simulink model "SIM_EXO_DAL_MN"  (R2021b)
settings: Solver=VariableStepAuto  StartTime=0.0  StopTime=60  FixedStep=0.0001  RelTol=1e-4
undefined symbols (not defined in the file): b, dq, q, X, Y, Z
libraries: sm_lib x47, nesl_utility x7
(part 20 of 24)

== matlab function SIM_EXO_DAL_MN/PD+g(DIN)/Gq ==
  data: q input; G output
function G = Gq(q)
%#codegen
q1 = q(1);
q2 = q(2);
q3 = q(3);
q4 = q(4);
q5 = q(5);
q6 = q(6);
%    This function was generated by the Symbolic Math Toolbox version 9.0.
%    02-Dec-2021 21:38:44

t2 = cos(q4);
t3 = cos(q5);
t4 = cos(q6);
t5 = sin(q4);
t6 = sin(q5);
t7 = sin(q6);
t8 = q1+q2;
t16 = 9.007199254740992e+15;
t9 = cos(t8);
t10 = sin(t8);
t19 = (q3.*t16)./9.007199254740992e+15;
t11 = t10.*7.742227997977903e+15;
t12 = t9.*4.602992943936994e+15;
t13 = t10.*4.602992943936994e+15;
t14 = t9.*7.742227997977903e+15;
t20 = cos(t19);
t21 = sin(t19);
t22 = t3.*t10.*1.11711378834605e-4;
t23 = t3.*t9.*1.878983903386652e-4;
t25 = t5.*t6.*t10.*1.878983903386652e-4;
t26 = t5.*t6.*t9.*3.16044842165395e-4;
t31 = t10.*3.412222012061753e-3;
t32 = t9.*5.313226374396773e-3;
t15 = -t13;
t17 = t11+t12;
t24 = -t22;
t27 = -t26;
t28 = t20.*7.38843356682345e-1;
t29 = t20.*2.61156643317655e-1;
t30 = t20.*4.392651260556773e-1;
t33 = -t31;
t34 = t20.*t23;
t35 = t3.*t10.*t20.*3.16044842165395e-4;
t36 = t3.*t9.*t20.*(-1.878983903386652e-4);
t38 = t5.*t6.*t9.*t20.*1.11711378834605e-4;
t39 = t20.*t25;
t41 = t5.*t6.*t10.*t20.*(-1.878983903386652e-4);
t44 = t2.*t16.*t21.*(t13-t14).*(-1.232595164407831e-32);
t46 = t5.*t16.*t21.*(t13-t14).*(-1.232595164407831e-32);
t47 = (t5.*t16.*t21.*(t13-t14))./8.112963841460668e+31;
t48 = t2.*t6.*t10.*t16.*t21.*4.082091644006594e-20;
t49 = t2.*t6.*t9.*t16.*t21.*2.426929178367519e-20;
t55 = t9.*t20.*1.796561051029836e-3;
t56 = t10.*t20.*3.021813293822463e-3;
t18 = t14+t15;
t37 = -t35;
t40 = -t38;
t42 = (t2.*t16.*t17.*t21)./8.112963841460668e+31;
t43 = (t5.*t16.*t17.*t21)./8.112963841460668e+31;
t50 = -t48;
t51 = -t49;
t52 = t28+2.61156643317655e-1;
t53 = t29+7.38843356682345e-1;
t54 = t30-4.392651260556773e-1;
t57 = -t55;
t58 = -t56;
t45 = -t43;
t59 = t9.*t52;
t60 = t9.*t53;
t61 = t10.*t52;
t62 = t10.*t53;
t63 = t9.*t54;
t64 = t10.*t54;
t65 = -t62;
t66 = -t64;
t67 = t61+t63;
t68 = t60+t64;
t74 = -t2.*(t62-t63);
t76 = -t5.*(t62-t63);
t84 = -t3.*(t5.*(t62-t63)+(t2.*t16.*t21.*(t13-t14))./8.112963841460668e+31);
t85 = -t6.*(t5.*(t62-t63)+(t2.*t16.*t21.*(t13-t14))./8.112963841460668e+31);
t86 = t3.*(t5.*(t62-t63)+(t2.*t16.*t21.*(t13-t14))./8.112963841460668e+31);
t69 = t63+t65;
t70 = t59+t66;
t71 = t2.*t68;
t72 = t3.*t67;
t73 = t5.*t68;
t78 = t6.*t67.*1.37594917755e-10;
t81 = t44+t76;
t83 = t47+t74;
t75 = t3.*t70;
t77 = t6.*t70;
t79 = t42+t73;
t80 = t45+t71;
t87 = t7.*(t43-t71).*(-1.31098465253029e-3);
t88 = t4.*(t43-t71).*(-7.125499486421585e-4);
t89 = t7.*(t43-t71).*1.31098465253029e-3;
t82 = t6.*t79;
t90 = t3.*t79.*1.37594917755e-10;
t93 = t75+t85;
t94 = t77+t86;
t91 = -t90;
t92 = t72+t82;
t95 = t4.*t92.*1.31098465253029e-3;
t96 = t7.*t92.*7.125499486421585e-4;
t97 = -t95;
t98 = -t96;
et1 = t16.*t21.*1.342380977036733e+41-t2.*t3.*t20.*4.732346230193865e+49-t2.*t6.*t20.*1.471195719231253e+56;
et2 = t4.*t5.*t20.*-2.450695940155113e+56+t5.*t7.*t20.*4.508911651294101e+56+t3.*t16.*t21.*1.403966899214815e+40;
et3 = t6.*t16.*t21.*-4.516093525807655e+33-t2.*t4.*t6.*t20.*4.508911651294101e+56-t2.*t6.*t7.*t20.*2.450695940155113e+56;
et4 = t2.*t4.*t16.*t21.*-1.390433427377147e+40+t3.*t4.*t16.*t21.*4.30286917447581e+40+t3.*t5.*t16.*t21.*2.684956660909679e+33+t2.*t7.*t16.*t21.*2.55818821842615e+40;
et5 = t3.*t7.*t16.*t21.*2.338707172024523e+40+t5.*t6.*t16.*t21.*8.347015526144078e+39+t4.*t5.*t6.*t16.*t21.*2.55818821842615e+40+t5.*t6.*t7.*t16.*t21.*1.390433427377147e+40;
et6 = t3.*(t46+t2.*(t62-t63)).*(-1.37594917755e-10);
et7 = t4.*(t5.*(t62-t63)+(t2.*t16.*t21.*(t13-t14))./8.112963841460668e+31).*(-7.125499486421585e-4);
et8 = t7.*(t5.*(t62-t63)+(t2.*t16.*t21.*(t13-t14))./8.112963841460668e+31).*1.31098465253029e-3;
et9 = t4.*t6.*(t46+t2.*(t62-t63)).*(-1.31098465253029e-3)-t6.*t7.*(t46+t2.*(t62-t63)).*7.125499486421585e-4;
et10 = t2.*t6.*t9.*(-1.878983903386652e-4);
et11 = t2.*t6.*t10.*(-3.16044842165395e-4);
et12 = t2.*t6.*t9.*t20.*1.878983903386652e-4;
et13 = t2.*t6.*t10.*t20.*(-1.11711378834605e-4)-t5.*t6.*t9.*t16.*t21.*4.082091644006594e-20;
et14 = t5.*t6.*t10.*t16.*t21.*2.426929178367519e-20;
et15 = t75.*(-1.37594917755e-10)-t6.*t9.*1.11711378834605e-4;
et16 = t6.*t10.*(-1.878983903386652e-4)+t5.*t34-t4.*t94.*1.31098465253029e-3;
et17 = t7.*t94.*(-7.125499486421585e-4);
et18 = t6.*(t5.*(t62-t63)+(t2.*t16.*t21.*(t13-t14))./8.112963841460668e+31).*1.37594917755e-10;
et19 = t3.*t5.*t9.*(-1.878983903386652e-4);
et20 = t3.*t5.*t10.*(-3.16044842165395e-4);
et21 = t6.*t9.*t20.*(-3.16044842165395e-4);
et22 = t6.*t10.*t20.*1.878983903386652e-4;
et23 = t3.*t5.*t10.*t20.*(-1.11711378834605e-4)+t2.*t3.*t9.*t16.*t21.*4.082091644006594e-20;
et24 = t2.*t3.*t10.*t16.*t21.*(-2.426929178367519e-20);
et25 = t4.*(t46+t2.*(t62-t63)).*(-1.31098465253029e-3)-t7.*(t46+t2.*(t62-t63)).*7.125499486421585e-4;
et26 = t4.*t93.*7.125499486421585e-4-t7.*t93.*1.31098465253029e-3;
mt1 = [t23+t24+t25+t27+t32+t33+t36+t37+t40+t41+t50+t51+t57+t58+t78+t88+t89+t91+t97+t98-3.963167671901972e+15.*sin(q1+atan(3.077527609784337e-1)).*1.978770022836862e-18;t23+t24+t25+t27+t32+t33+t36+t37+t40+t41+t50+t51+t57+t58+t78+t88+t89+t91+t97+t98];
mt2 = [(t13-t14).*(et1+et2+et3+et4+et5).*3.22801921778973e-76;et6+et7+et8+et9+et10+et11+et12+et13+et14;et15+et16+et17+et18+et19+et20+et21+et22+et23+et24;et25+et26];
G = [mt1;mt2];
